simulink model "Guarded_reference_for_structure"  (R2024b)
settings: Solver=ode3  StartTime=0.0  StopTime=60  FixedStep=4e-6  RelTol=1e-3  EnableMultiTasking=on
InitFcn:
  | dtime=4e-6;
  | Ts_step=1e-6;
  | run(fullfile(fileparts(get_param(bdroot,'FileName')),'TwoMass_Stage4_Params_5MW_Liu2024.m'));
  | run(fullfile(fileparts(get_param(bdroot,'FileName')),'TwoMass_Working_Experiment_Params.m'));
  | % Default disabled Vdc-reference profile interface (5 MW).
  | if ~exist('Vdc_ref_profile_keep','var') || ~Vdc_ref_profile_keep
  |     Vdc_ref_profile_ts = timeseries([1500;1500],[0;1e6]);
  | end
  | % IdealAvg copy-only electrical network sample time.
  | Ts_step=4e-6;
undefined symbols (not defined in the file): active_damping_scale, aero_release_delay_s, air_density, cp_beta_bp, cp_lambda_bp, cp_table, D_aero, D_g, D_sh, D_t, DiscIntNeverNeededParam, grid_frequency_hz, grid_voltage_peak_V, J_g, J_t, K_opt, K_sh, mppt_rated_blend_high_pu, mppt_rated_blend_low_pu, omega_m0, P_wt_rated, pitch_beta_ff_gain_deg_per_mps, pitch_beta_max_deg, pitch_enable, pitch_ff_start_wind_speed, pitch_integrator_initial_deg, pitch_ki_deg_per_rad, pitch_kp_deg_per_radps, pitch_rate_deg_per_s, rated_power_transition_duration_s, rated_power_transition_start_s, rotor_area, rotor_radius, stage4_aero_speed_damping_scale, stage4_ramp_duration_s, stage4_start_s, stage4_torque_ramp_Nmps, T_aero0, theta_tw_stage4_0, v_w0
libraries: spsCurrentMeasurementLib x12, spsSeriesRLCBranchLib x9, spsControlledVoltageSourceLib x6, spsVoltageMeasurementLib x6, simulink x3, powerlib_extras x2, spsControlledCurrentSourceLib x2, spsGroundLib x1, spsThreePhaseSourceLib x1, spsThreePhaseBreakerLib x1, sps_lib x1
(part 1 of 2)
settings Model: SimulationMode=accelerator  Creator=Administrator  LastModifiedBy=Lenovo
settings SolverCC: AlgebraicLoopSolver=TrustRegion
settings DataIOCC: LimitDataPoints=on  SaveFormat=Array  SignalLoggingSaveFormat=ModelDataLogs  SaveOutput=off  SignalLogging=off  SaveTime=off  ReturnWorkspaceOutputs=off
settings OptimizationCC: ExpressionDepthLimit=2147483647  LifeSpan=inf
settings DebuggingCC: UnderspecifiedInitializationDetection=Classic  MergeDetectMultiDrivingBlocksExec=none  SolverPrmCheckMsg=warning  FcnCallInpInsideContextMsg=warning  UnconnectedInputMsg=warning  UnconnectedOutputMsg=warning  UnconnectedLineMsg=warning  StateNameClashWarn=warning  SFUnexpectedBacktrackingDiag=warning  SFNoUnconditionalDefaultTransitionDiag=warning  SFExecutionAtInitializationDiag=none  ArithmeticOperatorsInVariantConditions=warning
settings HardwareCC: ProdBitPerPointer=32  ProdBitPerSizeT=32  ProdBitPerPtrDiffT=32  ProdLargestAtomicFloat=None  ProdIntDivRoundTo=Undefined  ProdEndianess=Unspecified  ProdWordSize=32  ProdHWDeviceType=32-bit Generic
settings ModelReferenceCC: EnableRefExpFcnMdlSchedulingChecks=on  PropagateSignalLabelsOutOfModel=off
settings SFSimCC: SimUseLocalCustomCode=off  CustomCodeUndefinedFunction=UseInterfaceOnly
settings RTWCC: RTWUseLocalCustomCode=off  GPUComputeCapability=3.5
settings CodeAppCC: StateflowObjectComments=on
settings GRTTargetCC: TargetLangStandard=C89/C90 (ANSI)
settings ConfigComp: CovMetricSettings=dw  CovSaveCumulativeToWorkspaceVar=on  CovSaveSingleToWorkspaceVar=on  CovExternalEMLEnable=off
settings SimscapeCC: SimscapeNormalizeSystem=off

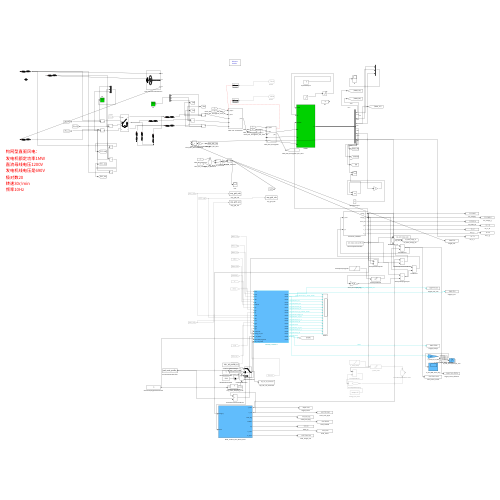
[thumbnail: Simulink's stored preview of the top-level diagram]
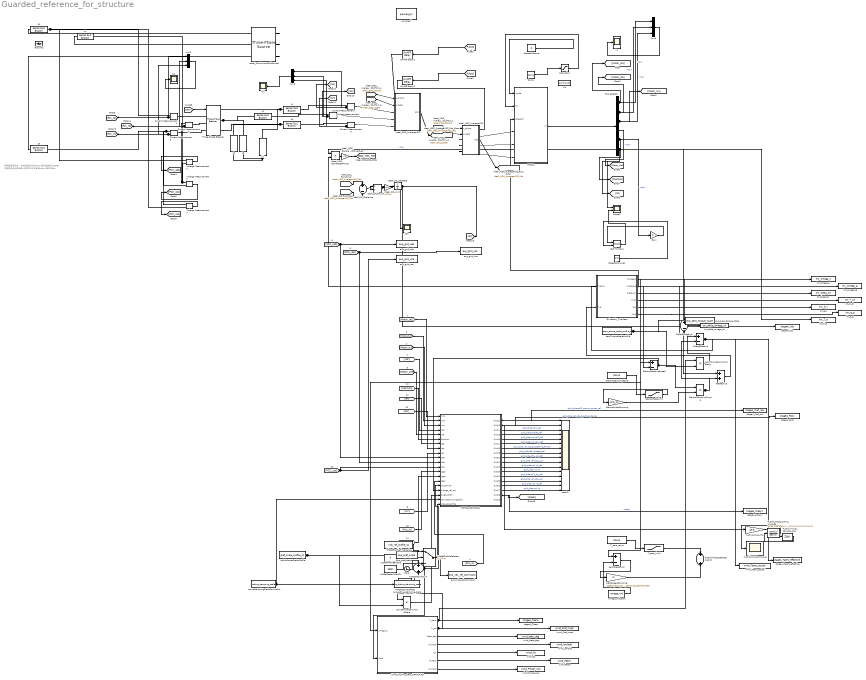
== system Guarded_reference_for_structure ==
  note: 构网型直驱风电：
      | 发电机额定功率1MW
      | 直流母线电压1200V
      | 发电机线电压是690V
      | 极对数20
      | 转速30r/min
      | 频率10Hz
  0speed1torque : Constant  Value=0
  0speed1torque1 : Constant  Value=2*pi
  ActiveDampingScaleCommand : Constant  Value=active_damping_scale
  ActivePowerCommandScale : Product  Inputs=**
  ActivePowerScaleProfile : FromWorkspace  VariableName=pref_scale_profile_ts  OutputAfterFinalValue=Holding final value
  AeroSpeedDamping : Gain  Gain=-stage4_aero_speed_damping_scale*D_aero
  AeroSpeedError : Sum  Inputs=+-
  AeroTorqueCommandScale : Product  Inputs=**
  AeroTorqueScaleProfile : FromWorkspace  VariableName=aero_torque_scale_profile_ts  OutputAfterFinalValue=Holding final value
  Bus Selector : BusSelector  OutputSignals=Statormeasurements.ia1,Statormeasurements.ib1,Statormeasurements.ic1,Mechanical.we,Mechanical.pos,Mechanical.Te
  Clock : Clock
  Current Measurement{,1..5} (6 alike) : spsCurrentMeasurementLib/Current Measurement  PhasorSimulation=off  OutputType=Complex  PSBequivalent=0
  DeltaOmega_sh : Sum  Inputs=+-
  Drivetrain_TwoMass : Subsystem
  Gain : Gain  Gain=2
  Ground1 : spsGroundLib/Ground  LConnTagsString=a
  HotStartClockOffset : Constant  Value=0
  HotStartClockSum : Sum
  Hz : Constant  Value=10*2*pi/20
  Ideal_ContinuousGridSource : spsThreePhaseSourceLib/Three-Phase Source  InternalConnection=Yg  VoltagePhases=off  Voltage=sqrt(3/2)*grid_voltage_peak_V  PhaseAngle=0  Voltage_phases=[25e3 25e3 25e3]/sqrt(3)  PhaseAngles_phases=[0 -120 +120]  Frequency=grid_frequency_hz  NonIdealSource=off  SpecifyImpedance=off  Resistance=0.8929  Inductance=16.58e-3  ShortCircuitLevel=100e6  BaseVoltage=25e3  XRratio=7  BusType=swing  Pref=10e3  Qref=0  Prefabc=[10e3, 10e3, 10e3]  Qrefabc=[0, 0, 0]  Qmin=-inf  Qmax=inf
  Ideal_DC_InvC : Gain  Gain=1/(0.3)
  Ideal_DC_Pbalance : Sum  Inputs=+-
  Ideal_DC_PoverUdc : Product  Inputs=*/
  Ideal_DC_UdcState : Integrator  InitialCondition=1500
  Ideal_GSC_AverageVSC : Subsystem
  Ideal_MSC_AverageVSC : Subsystem
  Ideal_MSC_GeneratedPower : Product  Inputs=**
  Ideal_MSC_GeneratedPowerSign : Gain  Gain=-1
  Iu : Scope
  Iu1 : Scope
  Iu2 : Scope
  L1 : spsSeriesRLCBranchLib/Series RLC Branch  LConnTagsString=__new0  RConnTagsString=__new0  BranchType=RL  Resistance=0.00047610000000000003  Inductance=4.5464201043630816e-05  SetiL0=off  InitialCurrent=0  Capacitance=2e-3  Setx0=off  InitialVoltage=0  Measurements=None
  L2 : spsSeriesRLCBranchLib/Series RLC Branch  LConnTagsString=__new0  RConnTagsString=__new0  BranchType=RL  Resistance=0.00047610000000000003  Inductance=4.5464201043630816e-05  SetiL0=off  InitialCurrent=0  Capacitance=2e-3  Setx0=off  InitialVoltage=0  Measurements=None
  L3 : spsSeriesRLCBranchLib/Series RLC Branch  LConnTagsString=__new0  RConnTagsString=__new0  BranchType=RL  Resistance=0.0019044000000000001  Inductance=7.5773668406051368e-05  SetiL0=off  InitialCurrent=0  Capacitance=2e-3  Setx0=off  InitialVoltage=0  Measurements=None
  L4 : spsSeriesRLCBranchLib/Series RLC Branch  LConnTagsString=__new0  RConnTagsString=__new0  BranchType=RL  Resistance=0.0019044000000000001  Inductance=7.5773668406051368e-05  SetiL0=off  InitialCurrent=0  Capacitance=2e-3  Setx0=off  InitialVoltage=0  Measurements=None
  L5 : spsSeriesRLCBranchLib/Series RLC Branch  LConnTagsString=__new0  RConnTagsString=__new0  BranchType=RL  Resistance=0.0019044000000000001  Inductance=7.5773668406051368e-05  SetiL0=off  InitialCurrent=0  Capacitance=2e-3  Setx0=off  InitialVoltage=0  Measurements=None
  L6 : spsSeriesRLCBranchLib/Series RLC Branch  LConnTagsString=__new0  RConnTagsString=__new0  BranchType=RL  Resistance=0.00047610000000000003  Inductance=4.5464201043630816e-05  SetiL0=off  InitialCurrent=0  Capacitance=2e-3  Setx0=off  InitialVoltage=0  Measurements=None
  L7 : spsSeriesRLCBranchLib/Series RLC Branch  LConnTagsString=__new0  RConnTagsString=__new0  BranchType=RC  Resistance=0.1  Inductance=0.00025  SetiL0=off  InitialCurrent=0  Capacitance=0.000275  Setx0=off  InitialVoltage=0  Measurements=None
  L8 : spsSeriesRLCBranchLib/Series RLC Branch  LConnTagsString=__new0  RConnTagsString=__new0  BranchType=RC  Resistance=0.1  Inductance=0.00025  SetiL0=off  InitialCurrent=0  Capacitance=0.000275  Setx0=off  InitialVoltage=0  Measurements=None
  L9 : spsSeriesRLCBranchLib/Series RLC Branch  LConnTagsString=__new0  RConnTagsString=__new0  BranchType=RC  Resistance=0.1  Inductance=0.00025  SetiL0=off  InitialCurrent=0  Capacitance=0.000275  Setx0=off  InitialVoltage=0  Measurements=None
  MOTOR_CONTROL1 : Subsystem  mask{Pref=5000000, Qref=0, ReferenceACVoltage=460, ReferenceDCVoltage=1500, DVCGainScale=1}
      mask prompts: Pref "Active Power"; Qref "Reactive Power"; ReferenceACVoltage "Reference AC Voltage"; ReferenceDCVoltage "Reference DC Voltage"; DVCGainScale "DVC Gain Scale"
  Math Function : Math  Operator=mod  SignedPower=on
  Mux1 : Mux  Inputs=3
  Mux3 : Mux  Inputs=3
  Mux5 : Mux  Inputs=3
  On/Off Delay1 : powerlib_extras/Control  Blocks/On//Off Delay  type_delay=On delay  delay=dtime  ic=0
  On/Off Delay2 : powerlib_extras/Control  Blocks/On//Off Delay  type_delay=On delay  delay=dtime  ic=0
  PMSM1 : Subsystem  mask{Rpass=1e2, Cpass=1e-6, Flux=8.640000000000001, Rs=0.0005, Lq=0.00105, Ld=0.00105, pairs=20, J=4960009.92001984, Bw=0.001}
  P_Grid_MW_20ms_Avg : Scope
  P_Grid_Paper_20ms_Average : DiscreteTransferFcn  Numerator=[0.05 0.05 0.05 0.05 0.05 0.05 0.05 0.05 0.05 0.05 0.05 0.05 0.05 0.05 0.05 0.05 0.05 0.05 0.05 0.05]  Denominator=[1 0 0 0 0 0 0 0 0 0 0 0 0 0 0 0 0 0 0 0]  SampleTime=0.001
  P_Grid_Visual_Sample_1ms : ZeroOrderHold  SampleTime=0.001
  P_Grid_W_to_MW : Gain  Gain=1e-6
  Ramp : simulink/Sources/Ramp  slope=1000  start=0.2  InitialOutput=0
  Saturation : Saturate  UpperLimit=9.55
  Scope1 : Scope  NumInputPorts=2
  StartupDampingFade : simulink/Sources/Ramp  slope=-0.5  start=10  InitialOutput=1
  StartupDampingTorque : Product  Inputs=**
  StartupExtraDamping : Gain  Gain=4*D_sh
  StartupFadeLimit : Saturate  UpperLimit=1  LowerLimit=0
  StartupRelativeSpeed : Sum  Inputs=+-
  T_aero_limit : Saturate  UpperLimit=(1+0.040000000000000001)*T_aero0  LowerLimit=0
  T_aero_ramp : simulink/Sources/Ramp  slope=stage4_torque_ramp_Nmps  start=stage4_start_s  InitialOutput=0
  TaeroEffective : Sum  Inputs=+-
  TaeroWithSpeedRestoration : Sum
  TeEffective : Sum
  Three-Phase Breaker : spsThreePhaseBreakerLib/Three-Phase Breaker  InitialState=open  SwitchA=on  SwitchB=on  SwitchC=on  SwitchTimes=[61.01 61.02]  External=on  BreakerResistance=0.0001  SnubberResistance=1e6  SnubberCapacitance=inf  Measurements=None
  Udc : Scope
  VdcRefDefault1500V : Constant  Value=1500
  VdcRefProfileEnable : Constant  Value=0
  VdcRefProfileSelector : Switch  Criteria=u2 ~= 0  Threshold=0.5  SaturateOnIntegerOverflow=off  InputSameDT=off
  VdcRefProfileTimeSeries : FromWorkspace  VariableName=Vdc_ref_profile_ts
  Voltage Measurement2 : spsVoltageMeasurementLib/Voltage Measurement  PhasorSimulation=off  OutputType=Complex  PSBequivalent=0
  Voltage Measurement3 : spsVoltageMeasurementLib/Voltage Measurement  PhasorSimulation=off  OutputType=Complex  PSBequivalent=0
  Voltage Measurement4 : spsVoltageMeasurementLib/Voltage Measurement  PhasorSimulation=off  OutputType=Complex  PSBequivalent=0
  Wind_Turbine_Aero_MPPT_Pitch : Subsystem
  exp_active_damping_scale : ToWorkspace  VariableName=exp_active_damping_scale  SaveFormat=Timeseries  SampleTime=-1
      settings: Decimation=1000
  exp_aero_torque_scale : ToWorkspace  VariableName=exp_aero_torque_scale  SaveFormat=Timeseries  SampleTime=-1
      settings: Decimation=1000
  exp_grid_uab : ToWorkspace  VariableName=exp_grid_uab  SaveFormat=Timeseries
      settings: Decimation=grid_frequency_log_decimation
  exp_grid_ubc : ToWorkspace  VariableName=exp_grid_ubc  SaveFormat=Timeseries
      settings: Decimation=grid_frequency_log_decimation
  exp_grid_uca : ToWorkspace  VariableName=exp_grid_uca  SaveFormat=Timeseries
      settings: Decimation=grid_frequency_log_decimation
  exp_pref_scale : ToWorkspace  VariableName=exp_pref_scale  SaveFormat=Timeseries  SampleTime=-1
      settings: Decimation=1000
  exp_vdc_ref_command : ToWorkspace  VariableName=exp_vdc_ref_command  SaveFormat=Structure With Time  SampleTime=-1
  omega_m0_aero : Constant  Value=omega_m0
  powergui : sps_lib/powergui  SimulationMode=Discrete  SampleTime=Ts_step  frequency=50  Iterations=50  frequencyindice=0  Pbase=5000000  ErrMax=1e-4  UnitsV=kV  UnitsW=MW  buscounter=0  FunctionMessages=off  echomessages=off  EnableUseOfTLC=off  CurrentSourceSwitches=off  DisableSnubberDevices=off  DisableRonSwitches=off  DisableVfSwitches=off  DisplayEquations=off  AutomaticDiscreteSolvers=off  SolverType=Tustin  Interpol=off  ExternalGateDelay=off  methode=off  Ts=0  x0status=blocks  SPID=off  SwTol=0  HookPort=off  NonlinearTolerance=1e-4  nMaxIteration=100  ContinueOnMaxIteration=off  RestoreLinks=warning  ResistiveCurrentMeasurement=off  Frange=[0:2:500]  Ylog=off  Xlog=on  ShowGrid=off  save=off  variable=ZData  structure=Iu1  ZoomFFT=off  StartTime=3.5  cycles=3  DisplayStyle=4  fundamental=50  FreqAxis=off  MaxFrequency=4000  frequencyindicesteady=1  RmsSteady=1  display=off
  stage4_Ppcc : ToWorkspace  VariableName=stage4_Ppcc  SaveFormat=Timeseries  SampleTime=-1
      settings: Decimation=mech_log_decimation
  stage4_PreSyn : ToWorkspace  VariableName=stage4_PreSyn  SaveFormat=Timeseries  SampleTime=-1
      settings: Decimation=mech_log_decimation
  stage4_Pref_raw : ToWorkspace  VariableName=stage4_Pref_raw  SaveFormat=Timeseries  SampleTime=-1
      settings: Decimation=mech_log_decimation
  stage4_Taero : ToWorkspace  VariableName=stage4_Taero  SaveFormat=Timeseries  SampleTime=-1
      settings: Decimation=mech_log_decimation
  stage4_Taero_effective : ToWorkspace  VariableName=stage4_Taero_effective  SaveFormat=Timeseries  SampleTime=-1
      settings: Decimation=mech_log_decimation
  stage4_Udc : ToWorkspace  VariableName=stage4_Udc  SaveFormat=Timeseries  SampleTime=-1
      settings: Decimation=mech_log_decimation
  tm_T_e : ToWorkspace  VariableName=tm_T_e  SaveFormat=Timeseries  SampleTime=-1
      settings: Decimation=mech_log_decimation
  tm_T_sh : ToWorkspace  VariableName=tm_T_sh  SaveFormat=Timeseries  SampleTime=-1
      settings: Decimation=mech_log_decimation
  tm_delta_omega_sh : ToWorkspace  VariableName=tm_delta_omega_sh  SaveFormat=Timeseries  SampleTime=-1
      settings: Decimation=mech_log_decimation
  tm_e_g : ToWorkspace  VariableName=tm_e_g  SaveFormat=Timeseries  SampleTime=-1
      settings: Decimation=mech_log_decimation
  tm_e_t : ToWorkspace  VariableName=tm_e_t  SaveFormat=Timeseries  SampleTime=-1
      settings: Decimation=mech_log_decimation
  tm_omega_g : ToWorkspace  VariableName=tm_omega_g  SaveFormat=Timeseries  SampleTime=-1
      settings: Decimation=mech_log_decimation
  tm_omega_t : ToWorkspace  VariableName=tm_omega_t  SaveFormat=Timeseries  SampleTime=-1
      settings: Decimation=mech_log_decimation
  tm_theta_tw : ToWorkspace  VariableName=tm_theta_tw  SaveFormat=Timeseries  SampleTime=-1
      settings: Decimation=mech_log_decimation
  watch2 : Scope  NumInputPorts=16
  wind_Cp : ToWorkspace  VariableName=wind_Cp  SaveFormat=Timeseries  SampleTime=-1
      settings: MaxDataPoints=200000  Decimation=1000
  wind_Paero : ToWorkspace  VariableName=wind_Paero  SaveFormat=Timeseries  SampleTime=-1
      settings: MaxDataPoints=200000  Decimation=1000
  wind_Pmppt_raw : ToWorkspace  VariableName=wind_Pmppt_raw  SaveFormat=Timeseries  SampleTime=-1
      settings: MaxDataPoints=200000  Decimation=1000
  wind_Pref_mppt : ToWorkspace  VariableName=wind_Pref_mppt  SaveFormat=Timeseries  SampleTime=-1
      settings: MaxDataPoints=200000  Decimation=1000
  wind_Taero_actual : ToWorkspace  VariableName=wind_Taero_actual  SaveFormat=Timeseries  SampleTime=-1
      settings: Decimation=mech_log_decimation
  wind_beta_deg : ToWorkspace  VariableName=wind_beta_deg  SaveFormat=Timeseries  SampleTime=-1
      settings: MaxDataPoints=200000  Decimation=1000
  wind_lambda : ToWorkspace  VariableName=wind_lambda  SaveFormat=Timeseries  SampleTime=-1
      settings: MaxDataPoints=200000  Decimation=1000
  tag scope: Ideal_GSC_AverageVSC_Pdc=global, Ideal_MSC_AverageVSC_Pdc=global, Ideal_MSC_Pdc=global
  wires:
  P_Grid_W_to_MW/1 -> P_Grid_Visual_Sample_1ms/1
  AeroTorqueCommandScale/1 -> TaeroEffective/1
  ActivePowerCommandScale/1 -> MOTOR_CONTROL1/18(P_ref_MPPT)
  ActiveDampingScaleCommand/1 -> exp_active_damping_scale/1, MOTOR_CONTROL1/19(ActiveDampingScale)
  AeroTorqueScaleProfile/1 -> AeroTorqueCommandScale/2, exp_aero_torque_scale/1
  ActivePowerScaleProfile/1 -> ActivePowerCommandScale/2, exp_pref_scale/1
  Wind_Turbine_Aero_MPPT_Pitch/7(P_mppt) -> wind_Pmppt_raw/1
  Wind_Turbine_Aero_MPPT_Pitch/6(P_aero) -> wind_Paero/1
  Wind_Turbine_Aero_MPPT_Pitch/5(Cp) -> wind_Cp/1
  Wind_Turbine_Aero_MPPT_Pitch/4(lambda) -> wind_lambda/1
  Wind_Turbine_Aero_MPPT_Pitch/3(beta_deg) -> wind_beta_deg/1
  Wind_Turbine_Aero_MPPT_Pitch/1(T_aero) -> stage4_Taero/1, AeroTorqueCommandScale/1
  Wind_Turbine_Aero_MPPT_Pitch/2(P_ref) -> wind_Pref_mppt/1, ActivePowerCommandScale/1
  TeEffective/1 -> Drivetrain_TwoMass/2(T_e)
  TaeroEffective/1 -> Drivetrain_TwoMass/1(T_aero), wind_Taero_actual/1, stage4_Taero_effective/1
  StartupDampingTorque/1 -> TeEffective/2, TaeroEffective/2
  StartupExtraDamping/1 -> StartupDampingTorque/2
  StartupRelativeSpeed/1 -> MOTOR_CONTROL1/17(omega_rel_ad), StartupDampingTorque/1
  StartupFadeLimit/1 -> StartupExtraDamping/1
  StartupDampingFade/1 -> StartupFadeLimit/1
  AeroSpeedDamping/1 -> TaeroWithSpeedRestoration/2
  AeroSpeedError/1 -> AeroSpeedDamping/1
  omega_m0_aero/1 -> AeroSpeedError/2
  T_aero_limit/1 -> TaeroWithSpeedRestoration/1
  T_aero_ramp/1 -> T_aero_limit/1
  Drivetrain_TwoMass/6(e_g) -> tm_e_g/1
  Drivetrain_TwoMass/5(e_t) -> tm_e_t/1
  Drivetrain_TwoMass/4(T_sh) -> tm_T_sh/1
  Drivetrain_TwoMass/3(theta_tw) -> tm_theta_tw/1
  Drivetrain_TwoMass/1(omega_t) -> Wind_Turbine_Aero_MPPT_Pitch/1(omega_t), AeroSpeedError/1, StartupRelativeSpeed/1, tm_omega_t/1, DeltaOmega_sh/1
  Drivetrain_TwoMass/2(omega_g) -> StartupRelativeSpeed/2, tm_omega_g/1, PMSM1/3(Speedin), DeltaOmega_sh/2, Ideal_MSC_GeneratedPower/2
  Current Measurement3/1 -> Mux3/3, [icn]
  Current Measurement2/1 -> [ibn], Mux3/2
  Current Measurement/1 -> [ian], Mux3/1
  Current Measurement5/1 -> [Pcc_ic], Mux1/3
  Current Measurement4/1 -> [Pcc_ib], Mux1/2
  Current Measurement1/1 -> [Pcc_ia], Mux1/1
  Mux1/1 -> Iu2/1
  [break] -> Three-Phase Breaker/1
  MOTOR_CONTROL1/17(Out28) -> stage4_PreSyn/1, [break]  "vector"
  [Pcc_ic] -> MOTOR_CONTROL1/15(Iggc)
  [Pcc_ib] -> MOTOR_CONTROL1/14(Iggb)
  [Pcc_ia] -> MOTOR_CONTROL1/13(Igga)
  Voltage Measurement3/1 -> [PCC_ubc]
  Voltage Measurement4/1 -> [PCC_uca]
  Voltage Measurement2/1 -> [PCC_uab]
  [ian] -> MOTOR_CONTROL1/7(Iga)
  [PCC_ubc] -> MOTOR_CONTROL1/11(Ubc), exp_grid_ubc/1
  [PCC_uca] -> MOTOR_CONTROL1/12(Uca), exp_grid_uca/1
  [ibn] -> MOTOR_CONTROL1/8(Igb)
  [PCC_uab] -> MOTOR_CONTROL1/10(Uab), exp_grid_uab/1
  [icn] -> MOTOR_CONTROL1/9(Igc)
  On/Off Delay1/1 -> ?
  [Pulse2] -> On/Off Delay1/1
  Mux3/1 -> Iu1/1
  [Motor_Ia1] -> MOTOR_CONTROL1/1(Ima)
  MOTOR_CONTROL1/8(Out19) -> watch2/8  "grid_side.ref.voltage_ref"
  MOTOR_CONTROL1/6(Out17) -> watch2/6  "grid_side.val.Uq1_ref"
  [vdc] -> MOTOR_CONTROL1/4(Udc)
  [Motor_Ic1] -> MOTOR_CONTROL1/3(Imc)
  [Position] -> MOTOR_CONTROL1/6(Position)
  MOTOR_CONTROL1/1(Out12) -> stage4_Pref_raw/1, watch2/1  "grid_side.ref.P_active_power_ref"
  MOTOR_CONTROL1/2(Out13) -> watch2/2, stage4_Ppcc/1, P_Grid_W_to_MW/1  "grid_side.val.pcc_P_active_Power"
  MOTOR_CONTROL1/11(Out22) -> watch2/11  "grid_side.val.Id_ref"
  MOTOR_CONTROL1/4(Out15) -> watch2/4  "grid_side.pf.thet_ref"
  MOTOR_CONTROL1/16(Out27) -> watch2/16  "grid_side.val.Iq"
  MOTOR_CONTROL1/3(Out14) -> watch2/3  "grid_side.pf.w_ref"
  MOTOR_CONTROL1/9(Out20) -> watch2/9  "grid_side.pf.U_od_ref"
  MOTOR_CONTROL1/10(Out21) -> watch2/10  "grid_side.val.pcc_u_d"
  MOTOR_CONTROL1/15(Out26) -> watch2/15  "grid_side.val.Iq_ref"
  [Motor_We] -> MOTOR_CONTROL1/5(We)
  MOTOR_CONTROL1/14(Out25) -> watch2/14  "grid_side.val.pcc_u_q"
  MOTOR_CONTROL1/5(Out16) -> watch2/5  "grid_side.val.Ud1_ref"
  MOTOR_CONTROL1/7(Out18) -> watch2/7  "grid_side.val.pcc_Q_reactive_Power"
  MOTOR_CONTROL1/13(Out24) -> watch2/13  "grid_side.pf.U_oq_ref"
  [Motor_Ib1] -> MOTOR_CONTROL1/2(Imb)
  MOTOR_CONTROL1/12(Out23) -> watch2/12  "grid_side.val.Id"
  Saturation/1 -> PMSM1/2(TL)
  0speed1torque1/1 -> Math Function/2
  0speed1torque/1 -> PMSM1/1(mode)
  Mux5/1 -> Iu/1
  Bus Selector/4 -> [Motor_We]  "<we>"
  Gain/1 -> Math Function/1
  Bus Selector/1 -> [Motor_Ia1], Mux5/1  "<ia1>"
  PMSM1/1(M) -> Bus Selector/1
  Bus Selector/2 -> [Motor_Ib1], Mux5/2  "<ib1>"
  Bus Selector/6 -> Scope1/1, [te], TeEffective/1, tm_T_e/1, Ideal_MSC_GeneratedPower/1  "<Te>"
  Ramp/1 -> Saturation/1
  Math Function/1 -> Scope1/2
  Bus Selector/3 -> [Motor_Ic1], Mux5/3  "<ic1>"
  Bus Selector/5 -> [Position], Gain/1  "<pos>"
  On/Off Delay2/1 -> ?
  [Pulse1] -> On/Off Delay2/1
  DeltaOmega_sh/1 -> tm_delta_omega_sh/1
  P_Grid_Visual_Sample_1ms/1 -> P_Grid_Paper_20ms_Average/1
  P_Grid_Paper_20ms_Average/1 -> P_Grid_MW_20ms_Avg/1
  VdcRefProfileTimeSeries/1 -> VdcRefProfileSelector/1
  VdcRefProfileEnable/1 -> VdcRefProfileSelector/2
  VdcRefDefault1500V/1 -> VdcRefProfileSelector/3
  VdcRefProfileSelector/1 -> MOTOR_CONTROL1/20(Vdc_ref_profile), exp_vdc_ref_command/1
  Clock/1 -> HotStartClockSum/1
  HotStartClockOffset/1 -> HotStartClockSum/2
  HotStartClockSum/1 -> MOTOR_CONTROL1/16(clockTime), Wind_Turbine_Aero_MPPT_Pitch/2(clock)
  Ideal_MSC_GeneratedPower/1 -> Ideal_MSC_GeneratedPowerSign/1
  Ideal_MSC_GeneratedPowerSign/1 -> [Ideal_MSC_Pdc]
  Ideal_GSC_AverageVSC/1(pdc) -> [Ideal_GSC_AverageVSC_Pdc]
  [Ideal_GSC_Ualpha] -> Ideal_GSC_AverageVSC/1(u_alpha)
  [Ideal_GSC_Ubeta] -> Ideal_GSC_AverageVSC/2(u_beta)
  Ideal_MSC_AverageVSC/1(pdc) -> [Ideal_MSC_AverageVSC_Pdc]
  [Ideal_MSC_Ualpha] -> Ideal_MSC_AverageVSC/1(u_alpha)
  [Ideal_MSC_Ubeta] -> Ideal_MSC_AverageVSC/2(u_beta)
  [Ideal_MSC_AverageVSC_Pdc] -> Ideal_DC_Pbalance/1
  [Ideal_GSC_AverageVSC_Pdc] -> Ideal_DC_Pbalance/2
  Ideal_DC_Pbalance/1 -> Ideal_DC_PoverUdc/1
  Ideal_DC_UdcState/1 -> Ideal_DC_PoverUdc/2, stage4_Udc/1, Udc/1, [vdc]
  Ideal_DC_PoverUdc/1 -> Ideal_DC_InvC/1
  Ideal_DC_InvC/1 -> Ideal_DC_UdcState/1
  connections:
  L1/RConn1 -- Current Measurement/RConn1
  Current Measurement2/RConn1 -- L2/RConn1
  Current Measurement3/RConn1 -- L6/RConn1
  Three-Phase Breaker/LConn3 -- Current Measurement5/LConn1
  Current Measurement4/LConn1 -- Three-Phase Breaker/LConn2
  Current Measurement1/LConn1 -- Three-Phase Breaker/LConn1
  L8/LConn1 -- Three-Phase Breaker/RConn2 -- L2/LConn1
  L1/LConn1 -- L7/LConn1 -- Three-Phase Breaker/RConn1
  L9/LConn1 -- Three-Phase Breaker/RConn3 -- L6/LConn1
  L7/RConn1 -- L8/RConn1 -- L9/RConn1
  Voltage Measurement4/LConn1 -- Voltage Measurement3/LConn2 -- Current Measurement5/RConn1 -- L5/RConn1
  Voltage Measurement3/LConn1 -- Voltage Measurement2/LConn2 -- Current Measurement4/RConn1 -- L4/RConn1
  Voltage Measurement2/LConn1 -- Voltage Measurement4/LConn2 -- Current Measurement1/RConn1 -- L3/RConn1
  Ideal_GSC_AverageVSC/LConn1 -- Current Measurement/LConn1
  Ideal_GSC_AverageVSC/LConn2 -- Current Measurement2/LConn1
  Ideal_GSC_AverageVSC/LConn3 -- Current Measurement3/LConn1
  Ideal_MSC_AverageVSC/LConn1 -- PMSM1/LConn1
  Ideal_MSC_AverageVSC/LConn2 -- PMSM1/LConn2
  Ideal_MSC_AverageVSC/LConn3 -- PMSM1/LConn3
  Ideal_ContinuousGridSource/RConn1 -- L3/LConn1
  Ideal_ContinuousGridSource/RConn2 -- L4/LConn1
  Ideal_ContinuousGridSource/RConn3 -- L5/LConn1

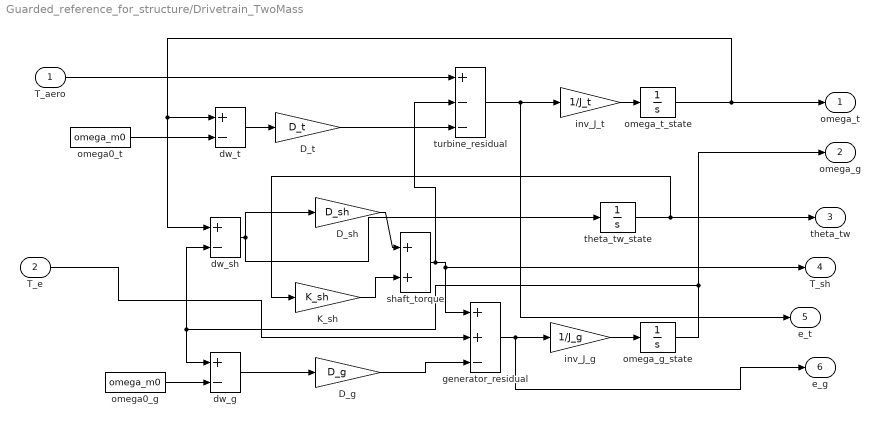
== system Guarded_reference_for_structure/Drivetrain_TwoMass ==
  T_aero : Inport
  T_e : Inport  Port=2
  D_g : Gain  Gain=D_g
  D_sh : Gain  Gain=D_sh
  D_t : Gain  Gain=D_t
  K_sh : Gain  Gain=K_sh
  dw_g : Sum  Inputs=+-
  dw_sh : Sum  Inputs=+-
  dw_t : Sum  Inputs=+-
  generator_residual : Sum  Inputs=++-
  inv_J_g : Gain  Gain=1/J_g
  inv_J_t : Gain  Gain=1/J_t
  omega0_g : Constant  Value=omega_m0
  omega0_t : Constant  Value=omega_m0
  omega_g_state : Integrator  InitialCondition=omega_m0
  omega_t_state : Integrator  InitialCondition=omega_m0
  shaft_torque : Sum
  theta_tw_state : Integrator  InitialCondition=theta_tw_stage4_0
  turbine_residual : Sum  Inputs=+--
  omega_t : Outport
  omega_g : Outport  Port=2
  theta_tw : Outport  Port=3
  T_sh : Outport  Port=4
  e_t : Outport  Port=5
  e_g : Outport  Port=6
  wires:
  inv_J_g/1 -> omega_g_state/1
  generator_residual/1 -> e_g/1, inv_J_g/1
  D_g/1 -> generator_residual/3
  T_e/1 -> generator_residual/2
  dw_g/1 -> D_g/1
  omega0_g/1 -> dw_g/2
  inv_J_t/1 -> omega_t_state/1
  turbine_residual/1 -> inv_J_t/1, e_t/1
  D_t/1 -> turbine_residual/3
  shaft_torque/1 -> turbine_residual/2, T_sh/1, generator_residual/1
  T_aero/1 -> turbine_residual/1
  dw_t/1 -> D_t/1
  omega0_t/1 -> dw_t/2
  K_sh/1 -> shaft_torque/2
  D_sh/1 -> shaft_torque/1
  theta_tw_state/1 -> K_sh/1, theta_tw/1
  dw_sh/1 -> theta_tw_state/1, D_sh/1
  omega_g_state/1 -> omega_g/1, dw_g/1, dw_sh/2
  omega_t_state/1 -> dw_t/1, dw_sh/1, omega_t/1

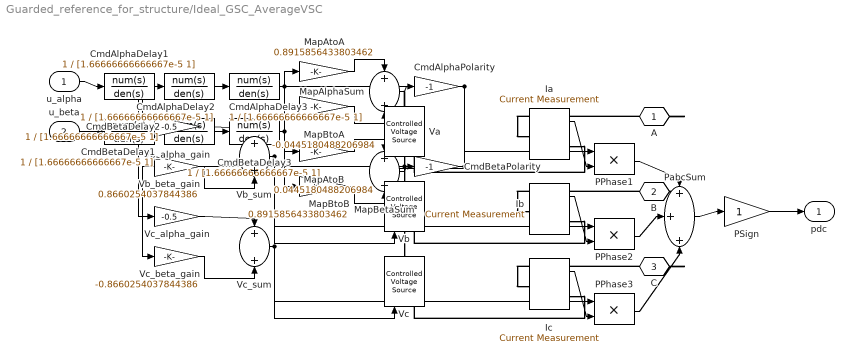
== system Guarded_reference_for_structure/Ideal_GSC_AverageVSC ==
  u_alpha : Inport
  u_beta : Inport  Port=2
  CmdAlphaDelay1 : TransferFcn  Numerator=1  Denominator=[1.66666666666667e-5 1]
  CmdAlphaDelay2 : TransferFcn  Numerator=1  Denominator=[1.66666666666667e-5 1]
  CmdAlphaDelay3 : TransferFcn  Numerator=1  Denominator=[1.66666666666667e-5 1]
  CmdAlphaPolarity : Gain  Gain=-1
  CmdBetaDelay1 : TransferFcn  Numerator=1  Denominator=[1.66666666666667e-5 1]
  CmdBetaDelay2 : TransferFcn  Numerator=1  Denominator=[1.66666666666667e-5 1]
  CmdBetaDelay3 : TransferFcn  Numerator=1  Denominator=[1.66666666666667e-5 1]
  CmdBetaPolarity : Gain  Gain=-1
  Ia : spsCurrentMeasurementLib/Current Measurement  PhasorSimulation=off  OutputType=Complex  PSBequivalent=0
  Ib : spsCurrentMeasurementLib/Current Measurement  PhasorSimulation=off  OutputType=Complex  PSBequivalent=0
  Ic : spsCurrentMeasurementLib/Current Measurement  PhasorSimulation=off  OutputType=Complex  PSBequivalent=0
  MapAlphaSum : Sum
  MapAtoA : Gain  Gain=0.8915856433803462
  MapAtoB : Gain  Gain=0.0445180488206984
  MapBetaSum : Sum
  MapBtoA : Gain  Gain=-0.0445180488206984
  MapBtoB : Gain  Gain=0.8915856433803462
  PPhase1 : Product  Inputs=**
  PPhase2 : Product  Inputs=**
  PPhase3 : Product  Inputs=**
  PSign : Gain
  PabcSum : Sum  Inputs=+++
  Va : spsControlledVoltageSourceLib/Controlled Voltage Source  Initialize=on  Source_Type=AC  Amplitude=0  Phase=0  Frequency=0  Measurements=None
  Vb : spsControlledVoltageSourceLib/Controlled Voltage Source  Initialize=on  Source_Type=AC  Amplitude=0  Phase=0  Frequency=0  Measurements=None
  Vb_alpha_gain : Gain  Gain=-0.5
  Vb_beta_gain : Gain  Gain=0.8660254037844386
  Vb_sum : Sum
  Vc : spsControlledVoltageSourceLib/Controlled Voltage Source  Initialize=on  Source_Type=AC  Amplitude=0  Phase=0  Frequency=0  Measurements=None
  Vc_alpha_gain : Gain  Gain=-0.5
  Vc_beta_gain : Gain  Gain=-0.8660254037844386
  Vc_sum : Sum
  A : PMIOPort  Side=Left
  B : PMIOPort  Port=2  Side=Left
  C : PMIOPort  Port=3  Side=Left
  pdc : Outport
  wires:
  u_alpha/1 -> CmdAlphaDelay1/1
  CmdAlphaDelay1/1 -> CmdAlphaDelay2/1
  CmdAlphaDelay2/1 -> CmdAlphaDelay3/1
  u_beta/1 -> CmdBetaDelay1/1
  CmdBetaDelay1/1 -> CmdBetaDelay2/1
  CmdBetaDelay2/1 -> CmdBetaDelay3/1
  CmdAlphaDelay3/1 -> MapAtoA/1, MapAtoB/1
  CmdBetaDelay3/1 -> MapBtoA/1, MapBtoB/1
  MapAtoA/1 -> MapAlphaSum/1
  MapBtoA/1 -> MapAlphaSum/2
  MapAtoB/1 -> MapBetaSum/1
  MapBtoB/1 -> MapBetaSum/2
  MapAlphaSum/1 -> CmdAlphaPolarity/1
  MapBetaSum/1 -> CmdBetaPolarity/1
  CmdAlphaPolarity/1 -> Va/1, Vb_alpha_gain/1, Vc_alpha_gain/1, PPhase1/1
  CmdBetaPolarity/1 -> Vb_beta_gain/1, Vc_beta_gain/1
  Vb_alpha_gain/1 -> Vb_sum/1
  Vb_beta_gain/1 -> Vb_sum/2
  Vb_sum/1 -> Vb/1, PPhase2/1
  Vc_alpha_gain/1 -> Vc_sum/1
  Vc_beta_gain/1 -> Vc_sum/2
  Vc_sum/1 -> Vc/1, PPhase3/1
  Ia/1 -> PPhase1/2
  Ib/1 -> PPhase2/2
  Ic/1 -> PPhase3/2
  PPhase1/1 -> PabcSum/1
  PPhase2/1 -> PabcSum/2
  PPhase3/1 -> PabcSum/3
  PabcSum/1 -> PSign/1
  PSign/1 -> pdc/1
  connections:
  A/RConn1 -- Ia/LConn1
  Ia/RConn1 -- Va/LConn1
  B/RConn1 -- Ib/LConn1
  Ib/RConn1 -- Vb/LConn1
  C/RConn1 -- Ic/LConn1
  Ic/RConn1 -- Vc/LConn1
  Vb/RConn1 -- Va/RConn1 -- Vc/RConn1

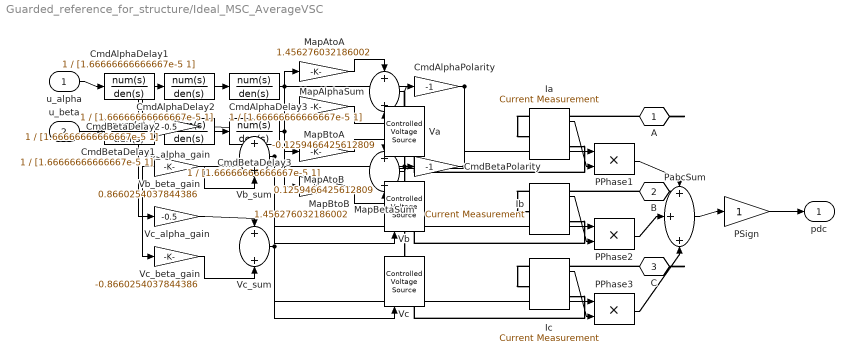
== system Guarded_reference_for_structure/Ideal_MSC_AverageVSC ==
  u_alpha : Inport
  u_beta : Inport  Port=2
  CmdAlphaDelay1 : TransferFcn  Numerator=1  Denominator=[1.66666666666667e-5 1]
  CmdAlphaDelay2 : TransferFcn  Numerator=1  Denominator=[1.66666666666667e-5 1]
  CmdAlphaDelay3 : TransferFcn  Numerator=1  Denominator=[1.66666666666667e-5 1]
  CmdAlphaPolarity : Gain  Gain=-1
  CmdBetaDelay1 : TransferFcn  Numerator=1  Denominator=[1.66666666666667e-5 1]
  CmdBetaDelay2 : TransferFcn  Numerator=1  Denominator=[1.66666666666667e-5 1]
  CmdBetaDelay3 : TransferFcn  Numerator=1  Denominator=[1.66666666666667e-5 1]
  CmdBetaPolarity : Gain  Gain=-1
  Ia : spsCurrentMeasurementLib/Current Measurement  PhasorSimulation=off  OutputType=Complex  PSBequivalent=0
  Ib : spsCurrentMeasurementLib/Current Measurement  PhasorSimulation=off  OutputType=Complex  PSBequivalent=0
  Ic : spsCurrentMeasurementLib/Current Measurement  PhasorSimulation=off  OutputType=Complex  PSBequivalent=0
  MapAlphaSum : Sum
  MapAtoA : Gain  Gain=1.456276032186002
  MapAtoB : Gain  Gain=0.1259466425612809
  MapBetaSum : Sum
  MapBtoA : Gain  Gain=-0.1259466425612809
  MapBtoB : Gain  Gain=1.456276032186002
  PPhase1 : Product  Inputs=**
  PPhase2 : Product  Inputs=**
  PPhase3 : Product  Inputs=**
  PSign : Gain
  PabcSum : Sum  Inputs=+++
  Va : spsControlledVoltageSourceLib/Controlled Voltage Source  Initialize=on  Source_Type=AC  Amplitude=0  Phase=0  Frequency=0  Measurements=None
  Vb : spsControlledVoltageSourceLib/Controlled Voltage Source  Initialize=on  Source_Type=AC  Amplitude=0  Phase=0  Frequency=0  Measurements=None
  Vb_alpha_gain : Gain  Gain=-0.5
  Vb_beta_gain : Gain  Gain=0.8660254037844386
  Vb_sum : Sum
  Vc : spsControlledVoltageSourceLib/Controlled Voltage Source  Initialize=on  Source_Type=AC  Amplitude=0  Phase=0  Frequency=0  Measurements=None
  Vc_alpha_gain : Gain  Gain=-0.5
  Vc_beta_gain : Gain  Gain=-0.8660254037844386
  Vc_sum : Sum
  A : PMIOPort  Side=Left
  B : PMIOPort  Port=2  Side=Left
  C : PMIOPort  Port=3  Side=Left
  pdc : Outport
  wires:
  u_alpha/1 -> CmdAlphaDelay1/1
  CmdAlphaDelay1/1 -> CmdAlphaDelay2/1
  CmdAlphaDelay2/1 -> CmdAlphaDelay3/1
  u_beta/1 -> CmdBetaDelay1/1
  CmdBetaDelay1/1 -> CmdBetaDelay2/1
  CmdBetaDelay2/1 -> CmdBetaDelay3/1
  CmdAlphaDelay3/1 -> MapAtoA/1, MapAtoB/1
  CmdBetaDelay3/1 -> MapBtoA/1, MapBtoB/1
  MapAtoA/1 -> MapAlphaSum/1
  MapBtoA/1 -> MapAlphaSum/2
  MapAtoB/1 -> MapBetaSum/1
  MapBtoB/1 -> MapBetaSum/2
  MapAlphaSum/1 -> CmdAlphaPolarity/1
  MapBetaSum/1 -> CmdBetaPolarity/1
  CmdAlphaPolarity/1 -> Va/1, Vb_alpha_gain/1, Vc_alpha_gain/1, PPhase1/1
  CmdBetaPolarity/1 -> Vb_beta_gain/1, Vc_beta_gain/1
  Vb_alpha_gain/1 -> Vb_sum/1
  Vb_beta_gain/1 -> Vb_sum/2
  Vb_sum/1 -> Vb/1, PPhase2/1
  Vc_alpha_gain/1 -> Vc_sum/1
  Vc_beta_gain/1 -> Vc_sum/2
  Vc_sum/1 -> Vc/1, PPhase3/1
  Ia/1 -> PPhase1/2
  Ib/1 -> PPhase2/2
  Ic/1 -> PPhase3/2
  PPhase1/1 -> PabcSum/1
  PPhase2/1 -> PabcSum/2
  PPhase3/1 -> PabcSum/3
  PabcSum/1 -> PSign/1
  PSign/1 -> pdc/1
  connections:
  A/RConn1 -- Ia/LConn1
  Ia/RConn1 -- Va/LConn1
  B/RConn1 -- Ib/LConn1
  Ib/RConn1 -- Vb/LConn1
  C/RConn1 -- Ic/LConn1
  Ic/RConn1 -- Vc/LConn1
  Vb/RConn1 -- Va/RConn1 -- Vc/RConn1

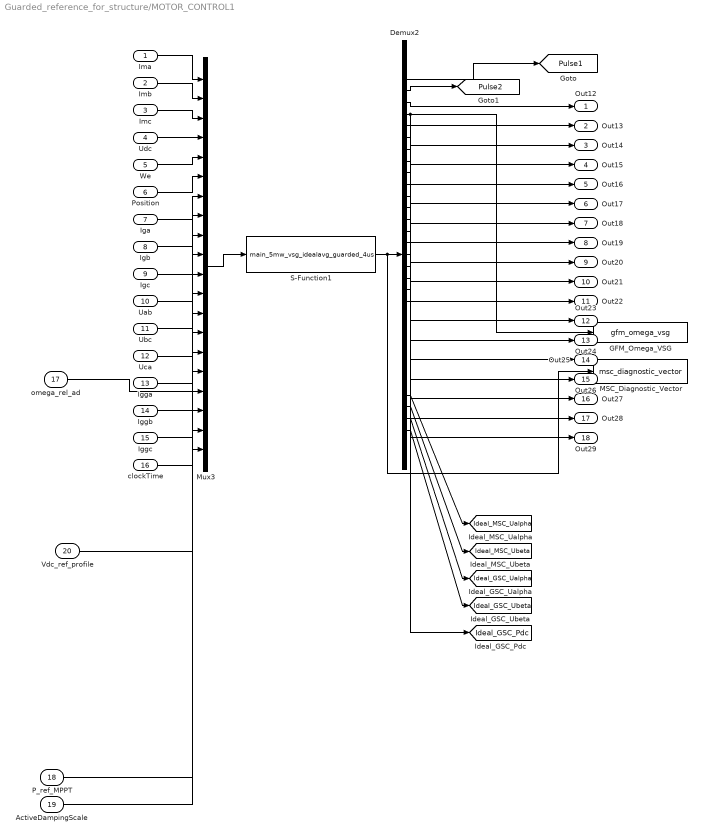
== system Guarded_reference_for_structure/MOTOR_CONTROL1 ==
  Ima : Inport
  Imb : Inport  Port=2
  Imc : Inport  Port=3
  Udc : Inport  Port=4
  We : Inport  Port=5
  Position : Inport  Port=6
  Iga : Inport  Port=7
  Igb : Inport  Port=8
  Igc : Inport  Port=9
  Uab : Inport  Port=10
  Ubc : Inport  Port=11
  Uca : Inport  Port=12
  Igga : Inport  Port=13
  Iggb : Inport  Port=14
  Iggc : Inport  Port=15
  clockTime : Inport  Port=16
  omega_rel_ad : Inport  Port=17
  P_ref_MPPT : Inport  Port=18
  ActiveDampingScale : Inport  Port=19
  Vdc_ref_profile : Inport  Port=20
  Demux2 : Demux  Outputs=[6 6 1 1 1 1 1 1 1 1 1 1 1 1 1 1 1 1 1 1 1 1 1 1 1 1 1 1 1 1 1]
      settings: DisplayOption=none
  GFM_Omega_VSG : ToWorkspace  VariableName=gfm_omega_vsg  SaveFormat=Timeseries  SampleTime=-1
      settings: MaxDataPoints=100000  Decimation=500
  MSC_Diagnostic_Vector : ToWorkspace  VariableName=msc_diagnostic_vector  SaveFormat=Timeseries  SampleTime=-1
      settings: MaxDataPoints=100000  Decimation=500
  Mux3 : Mux  Inputs=20
  S-Function1 : S-Function  FunctionName=main_5mw_vsg_idealavg_guarded_4us  Parameters=Pref Qref ReferenceACVoltage ReferenceDCVoltage DVCGainScale  SFunctionDeploymentMode=off  EnableBusSupport=off
  Out12 : Outport
  Out13 : Outport  Port=2
  Out14 : Outport  Port=3
  Out15 : Outport  Port=4
  Out16 : Outport  Port=5
  Out17 : Outport  Port=6
  Out18 : Outport  Port=7
  Out19 : Outport  Port=8
  Out20 : Outport  Port=9
  Out21 : Outport  Port=10
  Out22 : Outport  Port=11
  Out23 : Outport  Port=12
  Out24 : Outport  Port=13
  Out25 : Outport  Port=14
  Out26 : Outport  Port=15
  Out27 : Outport  Port=16
  Out28 : Outport  Port=17
  Out29 : Outport  Port=18
  tag scope: Ideal_GSC_Pdc=global, Ideal_GSC_Ualpha=global, Ideal_GSC_Ubeta=global, Ideal_MSC_Ualpha=global, Ideal_MSC_Ubeta=global, Pulse1=global, Pulse2=global
  wires:
  S-Function1/1 -> Demux2/1, MSC_Diagnostic_Vector/1
  Demux2/1 -> [Pulse1]
  Demux2/3 -> Out12/1
  Demux2/4 -> Out13/1, [Ideal_GSC_Pdc]
  Demux2/5 -> Out14/1, GFM_Omega_VSG/1
  Demux2/6 -> Out15/1
  Demux2/7 -> Out16/1
  Demux2/8 -> Out17/1
  Demux2/9 -> Out18/1
  Demux2/10 -> Out19/1
  Demux2/11 -> Out20/1
  Demux2/12 -> Out21/1
  Demux2/13 -> Out22/1
  Demux2/14 -> Out23/1
  Demux2/15 -> Out24/1
  Demux2/16 -> Out25/1
  Demux2/17 -> Out26/1
  Demux2/18 -> Out27/1
  Demux2/19 -> Out28/1
  Demux2/20 -> Out29/1
  Imb/1 -> Mux3/2
  Ima/1 -> Mux3/1
  Imc/1 -> Mux3/3
  We/1 -> Mux3/5
  Mux3/1 -> S-Function1/1
  Demux2/2 -> [Pulse2]
  Udc/1 -> Mux3/4
  Position/1 -> Mux3/6
  Uab/1 -> Mux3/10
  Ubc/1 -> Mux3/11
  Iga/1 -> Mux3/7
  Igb/1 -> Mux3/8
  Uca/1 -> Mux3/12
  Igc/1 -> Mux3/9
  Iggc/1 -> Mux3/15
  Iggb/1 -> Mux3/14
  Igga/1 -> Mux3/13
  clockTime/1 -> Mux3/16
  omega_rel_ad/1 -> Mux3/17
  P_ref_MPPT/1 -> Mux3/18
  ActiveDampingScale/1 -> Mux3/19
  Vdc_ref_profile/1 -> Mux3/20
  Demux2/28 -> [Ideal_MSC_Ualpha]
  Demux2/29 -> [Ideal_MSC_Ubeta]
  Demux2/30 -> [Ideal_GSC_Ualpha]
  Demux2/31 -> [Ideal_GSC_Ubeta]

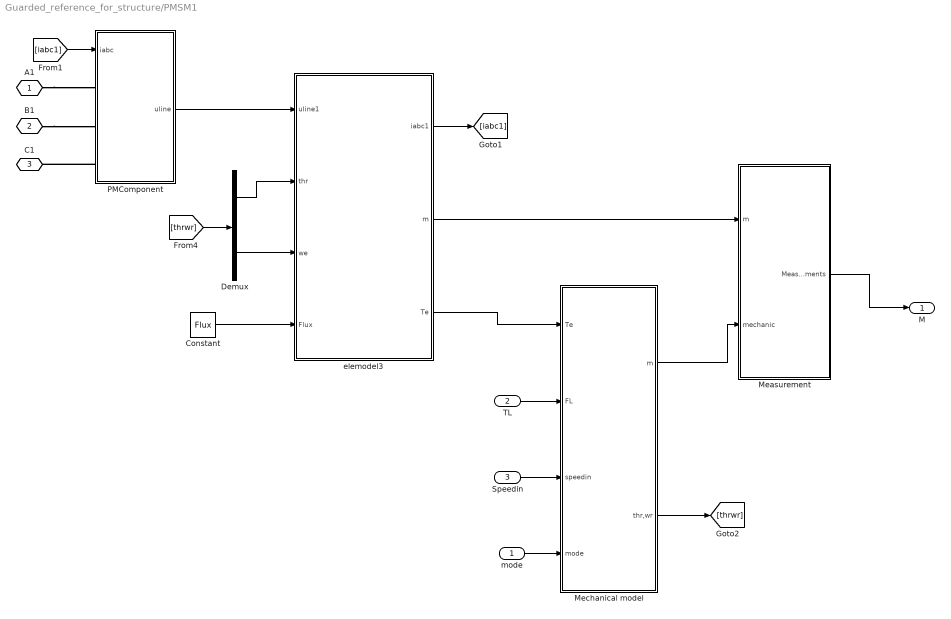
== system Guarded_reference_for_structure/PMSM1 ==
  mode : Inport
  TL : Inport  Port=2
  Speedin : Inport  Port=3
  Constant : Constant  Value=Flux
  Demux : Demux  Outputs=2
  Measurement : Subsystem
  Mechanical model : Subsystem
  PMComponent : Subsystem
  elemodel3 : Subsystem
  A1 : PMIOPort  Side=Left
  B1 : PMIOPort  Port=2  Side=Left
  C1 : PMIOPort  Port=3  Side=Left
  M : Outport
  wires:
  PMComponent/1(uline) -> elemodel3/1(uline1)
  Constant/1 -> elemodel3/4(Flux)
  Mechanical model/2(thr,wr) -> [thrwr]
  [thrwr] -> Demux/1
  Measurement/1(Measurements) -> M/1
  Mechanical model/1(m) -> Measurement/2(mechanic)
  TL/1 -> Mechanical model/2(FL)
  Speedin/1 -> Mechanical model/3(speedin)
  mode/1 -> Mechanical model/4(mode)
  elemodel3/3(Te) -> Mechanical model/1(Te)
  elemodel3/2(m) -> Measurement/1(m)
  Demux/1 -> elemodel3/2(thr)
  Demux/2 -> elemodel3/3(we)
  elemodel3/1(iabc1) -> [iabc1]
  [iabc1] -> PMComponent/1(iabc)
  connections:
  A1/RConn1 -- PMComponent/LConn1
  B1/RConn1 -- PMComponent/LConn2
  PMComponent/LConn3 -- C1/RConn1

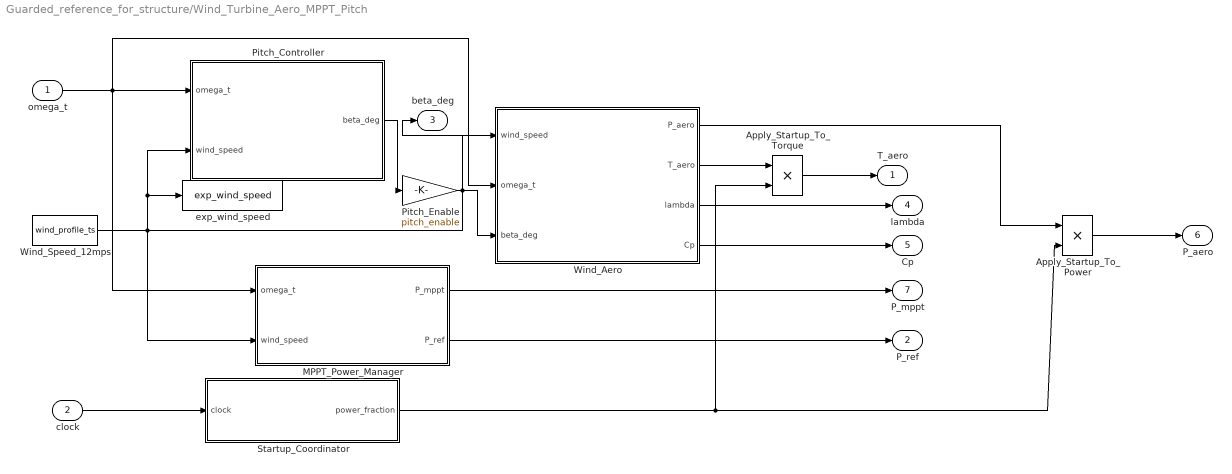
== system Guarded_reference_for_structure/Wind_Turbine_Aero_MPPT_Pitch ==
  omega_t : Inport
  clock : Inport  Port=2
  Apply_Startup_To_Power : Product  Inputs=**
  Apply_Startup_To_Torque : Product  Inputs=**
  MPPT_Power_Manager : Subsystem
  Pitch_Controller : Subsystem
  Pitch_Enable : Gain  Gain=pitch_enable
  Startup_Coordinator : Subsystem
  Wind_Aero : Subsystem
  Wind_Speed_12mps : FromWorkspace  VariableName=wind_profile_ts  OutputAfterFinalValue=Holding final value
  exp_wind_speed : ToWorkspace  VariableName=exp_wind_speed  SaveFormat=Timeseries  SampleTime=-1
      settings: Decimation=1000
  T_aero : Outport
  P_ref : Outport  Port=2
  beta_deg : Outport  Port=3
  lambda : Outport  Port=4
  Cp : Outport  Port=5
  P_aero : Outport  Port=6
  P_mppt : Outport  Port=7
  wires:
  omega_t/1 -> MPPT_Power_Manager/1(omega_t), Pitch_Controller/1(omega_t), Wind_Aero/2(omega_t)
  Wind_Speed_12mps/1 -> Pitch_Controller/2(wind_speed), exp_wind_speed/1, Wind_Aero/1(wind_speed), MPPT_Power_Manager/2(wind_speed)
  clock/1 -> Startup_Coordinator/1(clock)
  Wind_Aero/2(T_aero) -> Apply_Startup_To_Torque/1
  Startup_Coordinator/1(power_fraction) -> Apply_Startup_To_Power/2, Apply_Startup_To_Torque/2
  Wind_Aero/1(P_aero) -> Apply_Startup_To_Power/1
  Apply_Startup_To_Torque/1 -> T_aero/1
  MPPT_Power_Manager/2(P_ref) -> P_ref/1
  Wind_Aero/3(lambda) -> lambda/1
  Wind_Aero/4(Cp) -> Cp/1
  Apply_Startup_To_Power/1 -> P_aero/1
  MPPT_Power_Manager/1(P_mppt) -> P_mppt/1
  Pitch_Controller/1(beta_deg) -> Pitch_Enable/1
  Pitch_Enable/1 -> Wind_Aero/3(beta_deg), beta_deg/1

== system Guarded_reference_for_structure/PMSM1/Measurement ==
  m : Inport
  mechanic : Inport  Port=2
  Bus Creator : BusCreator  Inputs=8
  Bus Creator3 : BusCreator  Inputs=3
  Bus Creator5 : BusCreator  Inputs=2
  Demux : Demux  Outputs=[1,1,1,1,1,1,1,1]
  Demux1 : Demux  Outputs=[1,1,1]
  Measurements : Outport
  wires:
  m/1 -> Demux/1
  Bus Creator5/1 -> Measurements/1
  Demux/1 -> Bus Creator/1  "ia1"
  Demux/2 -> Bus Creator/2  "ib1"
  Demux/8 -> Bus Creator/8  "vc1"
  Demux/3 -> Bus Creator/3  "ic1"
  Bus Creator/1 -> Bus Creator5/1  "Statormeasurements"
  Bus Creator3/1 -> Bus Creator5/2  "Mechanical"
  ? -> ?  "fluxd"
  ? -> ?  "fluxq"
  mechanic/1 -> Demux1/1
  Demux1/1 -> Bus Creator3/1  "we"
  Demux1/2 -> Bus Creator3/2  "pos"
  Demux1/3 -> Bus Creator3/3  "Te"
  Demux/4 -> Bus Creator/4  "fluxd"
  Demux/5 -> Bus Creator/5  "fluxq"
  Demux/6 -> Bus Creator/6  "va1"
  Demux/7 -> Bus Creator/7  "vb1"

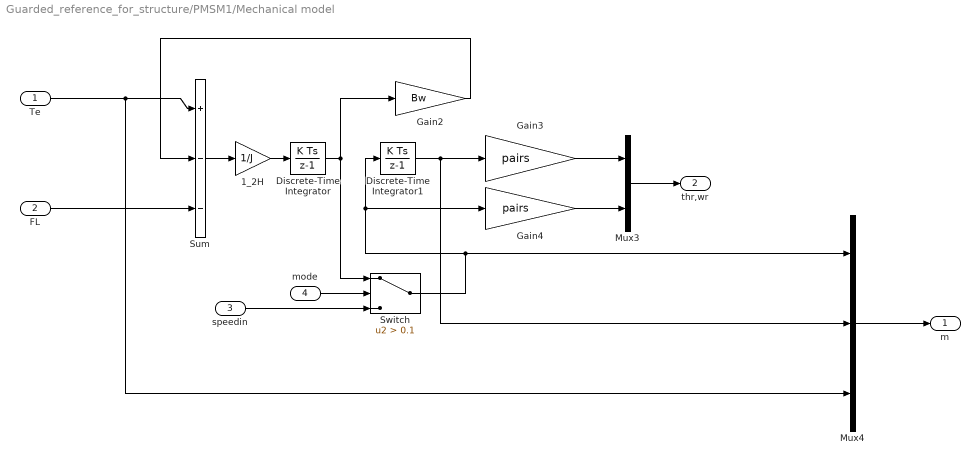
== system Guarded_reference_for_structure/PMSM1/Mechanical model ==
  Te : Inport
  FL : Inport  Port=2
  speedin : Inport  Port=3
  mode : Inport  Port=4
  1_2H : Gain  Gain=1/J  SaturateOnIntegerOverflow=on  OutDataTypeStr=Inherit: Same as input  ParamDataTypeStr=Inherit: Same as input
  Discrete-Time Integrator : DiscreteIntegrator  SampleTime=Ts_step  UpperSaturationLimit=1000000  LowerSaturationLimit=-1000000  ICPrevOutput=DiscIntNeverNeededParam  ICPrevScaledInput=DiscIntNeverNeededParam
  Discrete-Time Integrator1 : DiscreteIntegrator  SampleTime=Ts_step  ICPrevOutput=DiscIntNeverNeededParam  ICPrevScaledInput=DiscIntNeverNeededParam
  Gain2 : Gain  Gain=Bw
  Gain3 : Gain  Gain=pairs
  Gain4 : Gain  Gain=pairs
  Mux3 : Mux  Inputs=2
  Mux4 : Mux  Inputs=3
  Sum : Sum  Inputs=+--  InputSameDT=on  SaturateOnIntegerOverflow=on  OutDataTypeStr=Inherit: Same as first input
  Switch : Switch  Criteria=u2 > Threshold  Threshold=0.1  SaturateOnIntegerOverflow=off  InputSameDT=off
  m : Outport
  thr,wr : Outport  Port=2
  wires:
  Mux4/1 -> m/1
  Mux3/1 -> thr,wr/1
  Te/1 -> Sum/1, Mux4/3
  Sum/1 -> 1_2H/1
  Discrete-Time Integrator/1 -> Gain2/1, Switch/1
  Discrete-Time Integrator1/1 -> Gain3/1, Mux4/2
  1_2H/1 -> Discrete-Time Integrator/1
  Gain3/1 -> Mux3/1
  Gain4/1 -> Mux3/2
  mode/1 -> Switch/2
  speedin/1 -> Switch/3
  Switch/1 -> Discrete-Time Integrator1/1, Gain4/1, Mux4/1
  FL/1 -> Sum/3
  Gain2/1 -> Sum/2

== system Guarded_reference_for_structure/PMSM1/PMComponent ==
  iabc : Inport
  CURRENT INJECTION SYSTEM : Subsystem
  MEASUREMENT SYSTEM : Subsystem
  A1 : PMIOPort  Side=Left
  B1 : PMIOPort  Port=2  Side=Left
  C1 : PMIOPort  Port=3  Side=Left
  uline : Outport
  wires:
  iabc/1 -> CURRENT INJECTION SYSTEM/1(currents)
  MEASUREMENT SYSTEM/1(u_line) -> uline/1
  connections:
  B1/RConn1 -- MEASUREMENT SYSTEM/LConn2 -- CURRENT INJECTION SYSTEM/RConn2
  A1/RConn1 -- CURRENT INJECTION SYSTEM/RConn1 -- MEASUREMENT SYSTEM/LConn1
  MEASUREMENT SYSTEM/LConn3 -- C1/RConn1 -- CURRENT INJECTION SYSTEM/RConn3

== system Guarded_reference_for_structure/PMSM1/elemodel3 ==
  uline1 : Inport
  thr : Inport  Port=2
  we : Inport  Port=3
  Flux : Inport  Port=4
  Electromagnetic Force : Subsystem  AncestorBlock=|
      | spsSynchronousMachineModel/Continuous/Synchronous Machine
      | Continuous Model/Electromagnetic
      | Torque
  Machine Measurements : Mux  Inputs=[3,2,3]
  abc to dq : Subsystem  AncestorBlock="spsAsynchronousMachineModel/Continuous/abc to dq  transformation"
      mask Display: disp('abc2qd')
  dqtoabc : Subsystem
  iq,id : Subsystem  AncestorBlock=spsPMSynchronousMachineModel/Continuous/iq,id
  sin(thr),cos(thr)1 : Subsystem  TreatAsAtomicUnit=on
  iabc1 : Outport
  m : Outport  Port=2
  Te : Outport  Port=3
  wires:
  sin(thr),cos(thr)1/1(sin(thr),cos(thr)) -> abc to dq/2(sin,cos), dqtoabc/1(sincos)
  abc to dq/2(V_dq1) -> iq,id/1(vd1,vq1)
  Electromagnetic Force/1(F) -> Te/1
  uline1/1 -> abc to dq/1(uline)
  thr/1 -> sin(thr),cos(thr)1/1(thr)
  we/1 -> iq,id/2(we)
  Flux/1 -> iq,id/3(Flux), Electromagnetic Force/2(Flux)
  iq,id/1(id1,iq1) -> dqtoabc/2(dq), Electromagnetic Force/1(id1q1)
  dqtoabc/1(abc) -> iabc1/1, Machine Measurements/1
  Machine Measurements/1 -> m/1
  Electromagnetic Force/2(stator1flux) -> Machine Measurements/2
  abc to dq/1(statorvoltage) -> Machine Measurements/3

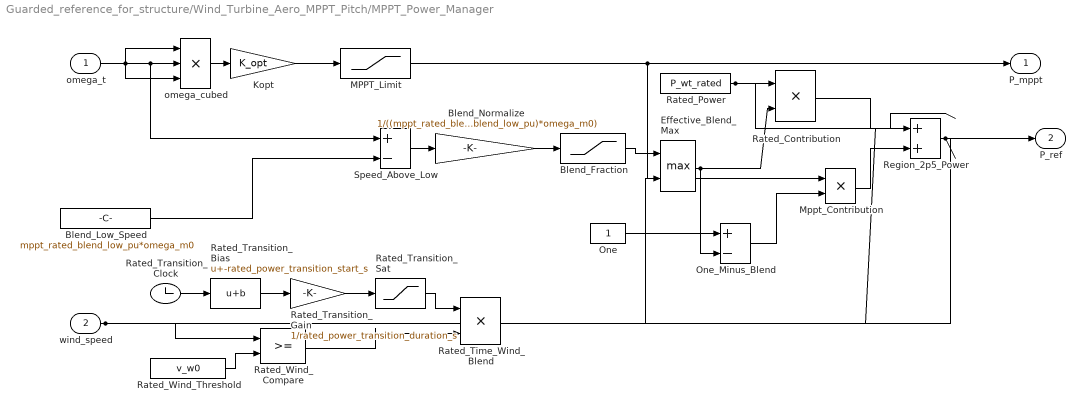
== system Guarded_reference_for_structure/Wind_Turbine_Aero_MPPT_Pitch/MPPT_Power_Manager ==
  omega_t : Inport
  wind_speed : Inport  Port=2
  Blend_Fraction : Saturate  UpperLimit=1  LowerLimit=0
  Blend_Low_Speed : Constant  Value=mppt_rated_blend_low_pu*omega_m0
  Blend_Normalize : Gain  Gain=1/((mppt_rated_blend_high_pu-mppt_rated_blend_low_pu)*omega_m0)
  Effective_Blend_Max : MinMax  Function=max  Inputs=2
  Kopt : Gain  Gain=K_opt
  MPPT_Limit : Saturate  UpperLimit=P_wt_rated  LowerLimit=0
  Mppt_Contribution : Product  Inputs=**
  One : Constant
  One_Minus_Blend : Sum  Inputs=+-
  Rated_Contribution : Product  Inputs=**
  Rated_Power : Constant  Value=P_wt_rated
  Rated_Time_Wind_Blend : Product  Inputs=**
  Rated_Transition_Bias : Bias  Bias=-rated_power_transition_start_s  SaturateOnIntegerOverflow=off
  Rated_Transition_Clock : Clock
  Rated_Transition_Gain : Gain  Gain=1/rated_power_transition_duration_s
  Rated_Transition_Sat : Saturate  UpperLimit=1  LowerLimit=0
  Rated_Wind_Compare : RelationalOperator  OutDataTypeStr=boolean  RndMeth=Simplest  InputSameDT=off
  Rated_Wind_Threshold : Constant  Value=v_w0
  Region_2p5_Power : Sum
  Speed_Above_Low : Sum  Inputs=+-
  omega_cubed : Product  Inputs=***
  P_mppt : Outport
  P_ref : Outport  Port=2
  wires:
  omega_t/1 -> omega_cubed/2, Speed_Above_Low/1, omega_cubed/1, omega_cubed/3
  omega_cubed/1 -> Kopt/1
  Kopt/1 -> MPPT_Limit/1
  MPPT_Limit/1 -> P_mppt/1, Mppt_Contribution/1
  Blend_Low_Speed/1 -> Speed_Above_Low/2
  Speed_Above_Low/1 -> Blend_Normalize/1
  Blend_Normalize/1 -> Blend_Fraction/1
  One/1 -> One_Minus_Blend/1
  One_Minus_Blend/1 -> Mppt_Contribution/2
  Rated_Contribution/1 -> Region_2p5_Power/1
  Mppt_Contribution/1 -> Region_2p5_Power/2
  wind_speed/1 -> Rated_Wind_Compare/1
  Rated_Power/1 -> Rated_Contribution/1
  Region_2p5_Power/1 -> P_ref/1
  Rated_Transition_Clock/1 -> Rated_Transition_Bias/1
  Rated_Transition_Bias/1 -> Rated_Transition_Gain/1
  Rated_Transition_Gain/1 -> Rated_Transition_Sat/1
  Rated_Wind_Threshold/1 -> Rated_Wind_Compare/2
  Rated_Transition_Sat/1 -> Rated_Time_Wind_Blend/1
  Rated_Wind_Compare/1 -> Rated_Time_Wind_Blend/2
  Blend_Fraction/1 -> Effective_Blend_Max/1
  Rated_Time_Wind_Blend/1 -> Effective_Blend_Max/2
  Effective_Blend_Max/1 -> Rated_Contribution/2, One_Minus_Blend/2

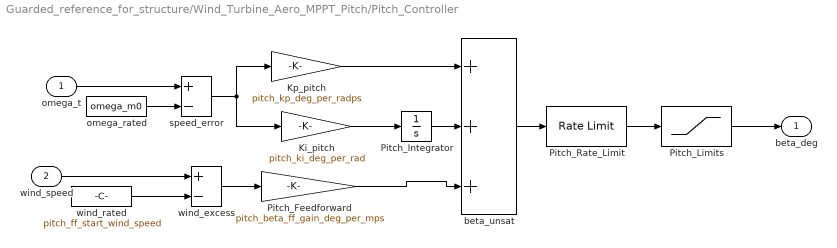
== system Guarded_reference_for_structure/Wind_Turbine_Aero_MPPT_Pitch/Pitch_Controller ==
  omega_t : Inport
  wind_speed : Inport  Port=2
  Ki_pitch : Gain  Gain=pitch_ki_deg_per_rad
  Kp_pitch : Gain  Gain=pitch_kp_deg_per_radps
  Pitch_Feedforward : Gain  Gain=pitch_beta_ff_gain_deg_per_mps
  Pitch_Integrator : Integrator  InitialCondition=pitch_integrator_initial_deg  LimitOutput=on  UpperSaturationLimit=pitch_beta_max_deg  LowerSaturationLimit=0
  Pitch_Limits : Saturate  UpperLimit=pitch_beta_max_deg  LowerLimit=0
  Pitch_Rate_Limit : RateLimiter  RisingSlewLimit=pitch_rate_deg_per_s  FallingSlewLimit=-pitch_rate_deg_per_s  SampleTimeMode=inherited
  beta_unsat : Sum  Inputs=+++
  omega_rated : Constant  Value=omega_m0
  speed_error : Sum  Inputs=+-
  wind_excess : Sum  Inputs=+-
  wind_rated : Constant  Value=pitch_ff_start_wind_speed
  beta_deg : Outport
  wires:
  omega_t/1 -> speed_error/1
  omega_rated/1 -> speed_error/2
  speed_error/1 -> Kp_pitch/1, Ki_pitch/1
  Ki_pitch/1 -> Pitch_Integrator/1
  wind_speed/1 -> wind_excess/1
  wind_rated/1 -> wind_excess/2
  wind_excess/1 -> Pitch_Feedforward/1
  Kp_pitch/1 -> beta_unsat/1
  Pitch_Integrator/1 -> beta_unsat/2
  beta_unsat/1 -> Pitch_Rate_Limit/1
  Pitch_Rate_Limit/1 -> Pitch_Limits/1
  Pitch_Limits/1 -> beta_deg/1
  ? -> ?
  ? -> ?
  Pitch_Feedforward/1 -> beta_unsat/3

== system Guarded_reference_for_structure/Wind_Turbine_Aero_MPPT_Pitch/Startup_Coordinator ==
  clock : Inport
  elapsed : Sum  Inputs=+-
  fraction_limits : Saturate  UpperLimit=1  LowerLimit=0
  release_time : Constant  Value=stage4_start_s+aero_release_delay_s
  to_fraction : Gain  Gain=1/stage4_ramp_duration_s
  power_fraction : Outport
  wires:
  clock/1 -> elapsed/1
  release_time/1 -> elapsed/2
  elapsed/1 -> to_fraction/1
  to_fraction/1 -> fraction_limits/1
  fraction_limits/1 -> power_fraction/1

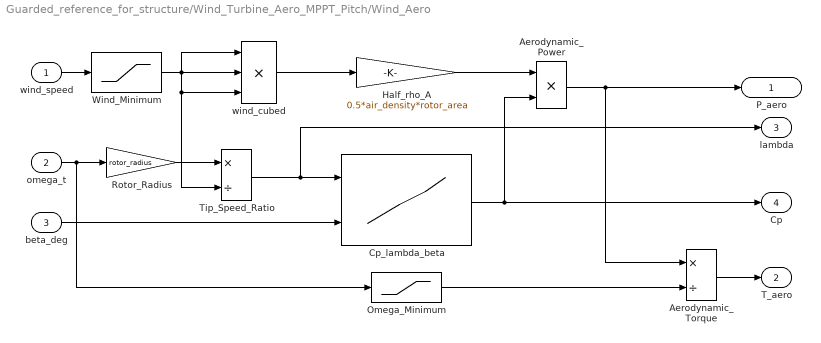
== system Guarded_reference_for_structure/Wind_Turbine_Aero_MPPT_Pitch/Wind_Aero ==
  wind_speed : Inport
  omega_t : Inport  Port=2
  beta_deg : Inport  Port=3
  Aerodynamic_Power : Product  Inputs=**
  Aerodynamic_Torque : Product  Inputs=*/
  Cp_lambda_beta : Lookup_n-D  BreakpointsForDimension1=cp_lambda_bp  BreakpointsForDimension2=cp_beta_bp  Table=cp_table  InternalRulePriority=Speed  RndMeth=Simplest
      settings: InputPortMap=u0,u1
  Half_rho_A : Gain  Gain=0.5*air_density*rotor_area
  Omega_Minimum : Saturate  UpperLimit=3  LowerLimit=0.2
  Rotor_Radius : Gain  Gain=rotor_radius
  Tip_Speed_Ratio : Product  Inputs=*/
  Wind_Minimum : Saturate  UpperLimit=60  LowerLimit=0.5
  wind_cubed : Product  Inputs=***
  P_aero : Outport
  T_aero : Outport  Port=2
  lambda : Outport  Port=3
  Cp : Outport  Port=4
  wires:
  wind_speed/1 -> Wind_Minimum/1
  Wind_Minimum/1 -> Tip_Speed_Ratio/2, wind_cubed/3, wind_cubed/2, wind_cubed/1
  omega_t/1 -> Rotor_Radius/1, Omega_Minimum/1
  Rotor_Radius/1 -> Tip_Speed_Ratio/1
  Tip_Speed_Ratio/1 -> lambda/1, Cp_lambda_beta/1
  beta_deg/1 -> Cp_lambda_beta/2
  wind_cubed/1 -> Half_rho_A/1
  Half_rho_A/1 -> Aerodynamic_Power/1
  Cp_lambda_beta/1 -> Cp/1, Aerodynamic_Power/2
  Aerodynamic_Power/1 -> P_aero/1, Aerodynamic_Torque/1
  Omega_Minimum/1 -> Aerodynamic_Torque/2
  Aerodynamic_Torque/1 -> T_aero/1

== system Guarded_reference_for_structure/PMSM1/PMComponent/CURRENT INJECTION SYSTEM ==
  currents : Inport
  Controlled Current Source : spsControlledCurrentSourceLib/Controlled Current Source  Initialize=on  Source_Type=AC  Amplitude=0  Phase=0  Frequency=0  Measurements=None
  Controlled Current Source1 : spsControlledCurrentSourceLib/Controlled Current Source  Initialize=on  Source_Type=AC  Amplitude=0  Phase=0  Frequency=0  Measurements=None
  Demux : Demux  Outputs=2
  Selector : Selector  InputPortWidth=3  IndexOptions=Index vector (dialog)  Indices=1:2  OutputSizes=1
  A1 : PMIOPort  Side=Right
  B1 : PMIOPort  Port=2  Side=Right
  C1 : PMIOPort  Port=3  Side=Right
  wires:
  Demux/1 -> Controlled Current Source/1
  Demux/2 -> Controlled Current Source1/1
  currents/1 -> Selector/1
  Selector/1 -> Demux/1
  connections:
  Controlled Current Source/LConn1 -- A1/RConn1
  Controlled Current Source1/LConn1 -- B1/RConn1
  Controlled Current Source/RConn1 -- Controlled Current Source1/RConn1 -- C1/RConn1

== system Guarded_reference_for_structure/PMSM1/PMComponent/MEASUREMENT SYSTEM ==
  Mux : Mux  Inputs=3
  V_AB : spsVoltageMeasurementLib/Voltage Measurement  PhasorSimulation=off  OutputType=Complex  PSBequivalent=0
  V_BC : spsVoltageMeasurementLib/Voltage Measurement  PhasorSimulation=off  OutputType=Complex  PSBequivalent=0
  V_CA : spsVoltageMeasurementLib/Voltage Measurement  PhasorSimulation=off  OutputType=Complex  PSBequivalent=0
  A1 : PMIOPort  Side=Left
  B1 : PMIOPort  Port=2  Side=Left
  C1 : PMIOPort  Port=3  Side=Left
  u_line : Outport
  wires:
  Mux/1 -> u_line/1
  V_BC/1 -> Mux/2
  V_AB/1 -> Mux/1
  V_CA/1 -> Mux/3
  connections:
  V_AB/LConn1 -- A1/RConn1 -- V_CA/LConn2
  V_BC/LConn2 -- C1/RConn1 -- V_CA/LConn1
  V_BC/LConn1 -- V_AB/LConn2 -- B1/RConn1

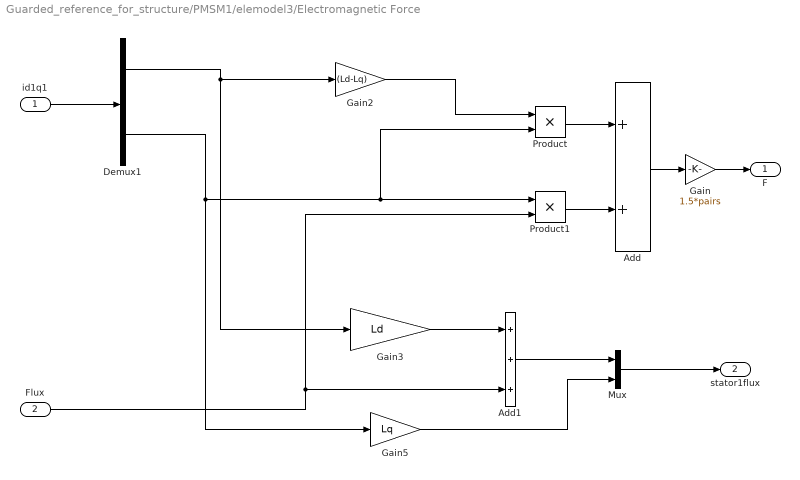
== system Guarded_reference_for_structure/PMSM1/elemodel3/Electromagnetic Force ==
  id1q1 : Inport
  Flux : Inport  Port=2
  Add : Sum
  Add1 : Sum  Inputs=+++
  Demux1 : Demux  Outputs=2
  Gain : Gain  Gain=1.5*pairs
  Gain2 : Gain  Gain=(Ld-Lq)
  Gain3 : Gain  Gain=Ld
  Gain5 : Gain  Gain=Lq
  Mux : Mux  Inputs=2
  Product : Product  RndMeth=Zero
  Product1 : Product  RndMeth=Zero
  F : Outport
  stator1flux : Outport  Port=2
  wires:
  id1q1/1 -> Demux1/1
  Add/1 -> Gain/1
  Product/1 -> Add/1
  Product1/1 -> Add/2
  Gain/1 -> F/1
  Gain3/1 -> Add1/1
  Add1/1 -> Mux/1
  Mux/1 -> stator1flux/1
  Flux/1 -> Product1/2, Add1/3
  Demux1/2 -> Product1/1, Product/2, Gain5/1
  Demux1/1 -> Gain2/1, Gain3/1
  Gain2/1 -> Product/1
  Gain5/1 -> Mux/2
